simulink library "halin"  (R2021b)
settings: Solver=VariableStepAuto  StartTime=0.0  StopTime=10.0  RelTol=1e-3
undefined symbols (not defined in the file): KHAL_CAN1ABM1E2E_flg, KHAL_CAN1EPB1E2E_flg, KHAL_CAN1EPS1E2E_flg, KHAL_CAN1ESC1E2E_flg, KHAL_CAN1ESC5E2E_flg, KHAL_CAN3BMS1E2E_flg, KHAL_CAN3BMS6E2E_flg, KHAL_CAN3CCU1E2E_flg, KHAL_CAN3CCU2E2E_flg, KHAL_CAN3MCUNF1E2E_flg, KHAL_CAN3MCUNR1E2E_flg, KHAL_CAN3Shifter1E2E_flg, KHAL_CAN3Shifter2E2E_flg, KHAL_CAN6FCM2E2E_flg, KHAL_CAN6FCM4E2E_flg, TRUE
libraries: simulink x645, FVT_lib x207, hcu_lib x59
(part 17 of 23)

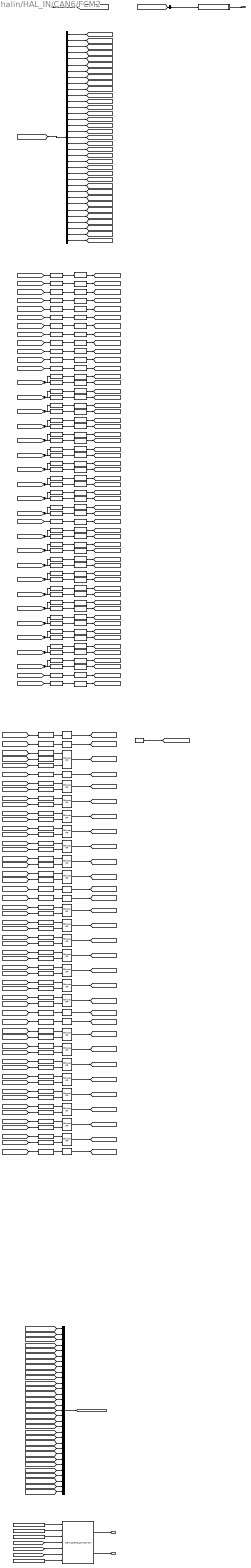
== system halin/HAL_IN/CAN6/FCM2 ==
  DT_CAN6_SG_FCM2 : Inport
  0x55 : Constant  Value=0x55
  0xEB : Constant  Value=0xEB
  ADBVehDst1Val : Subsystem
  BitwiseAND{,1..54} (55 alike) : simulink/Logic and Bit Operations/Bitwise Operator  logicop=AND  UseBitMask=on  BitMask=0xFF  BitMaskRealWorld=Stored Integer
  BitwiseOR{,1,3,11..12,20..21,30} (8 alike) : simulink/Logic and Bit Operations/Bitwise Operator  logicop=OR  UseBitMask=off  BitMask=bin2dec('11011001')  BitMaskRealWorld=Stored Integer
  BitwiseOR{4..10,13..19,22..29} (22 alike) : simulink/Logic and Bit Operations/Bitwise Operator  logicop=OR  UseBitMask=off  NumInputPorts=2  BitMask=bin2dec('11011001')  BitMaskRealWorld=Stored Integer
  BitwiseOR2 : simulink/Logic and Bit Operations/Bitwise Operator  logicop=OR  UseBitMask=off  NumInputPorts=3  BitMask=bin2dec('11011001')  BitMaskRealWorld=Stored Integer
  DDM_CS&RC_Comparison : FVT_lib/hal/DDM_CS&RC_Comparison  MsgCycleTime=50
  Data Type Conversion{,1..54} (55 alike) : DataTypeConversion  OutDataTypeStr=uint8
  KHAL_CAN6FCM2E2E_flg : Constant  Value=KHAL_CAN6FCM2E2E_flg
  LeftShift : ArithShift  BitShiftNumber=6  BitShiftDirection=Left
  LeftShift{1,3,5,7,9,11,13..14} (8 alike) : ArithShift  BitShiftDirection=Left
  LeftShift{2,4,6,8,10} (5 alike) : ArithShift  BitShiftNumber=4  BitShiftDirection=Left
  LeftShift12 : ArithShift  BitShiftNumber=2  BitShiftDirection=Left
  MessageRollingCounter : FVT_lib/hal/MessageRollingCounter  CounterMAX=14  task_time_ms=5  msg_time_ms=50
  Mux : Mux  Inputs=31
  RightShift : ArithShift  BitShiftNumber=3
  RightShift1 : ArithShift  BitShiftNumber=-5
  RightShift10 : ArithShift  BitShiftNumber=1
  RightShift11 : ArithShift  BitShiftNumber=-7
  RightShift12 : ArithShift  BitShiftNumber=3
  RightShift13 : ArithShift  BitShiftNumber=-5
  RightShift14 : ArithShift  BitShiftNumber=5
  RightShift15 : ArithShift  BitShiftNumber=-3
  RightShift16 : ArithShift  BitShiftNumber=7
  RightShift17 : ArithShift  BitShiftNumber=-1
  RightShift18 : ArithShift  BitShiftNumber=1
  RightShift19 : ArithShift  BitShiftNumber=-7
  RightShift2 : ArithShift  BitShiftNumber=1
  RightShift20 : ArithShift  BitShiftNumber=4
  RightShift21 : ArithShift  BitShiftNumber=-4
  RightShift22 : ArithShift  BitShiftNumber=2
  RightShift23 : ArithShift  BitShiftNumber=-6
  RightShift24 : ArithShift  BitShiftNumber=4
  RightShift25 : ArithShift  BitShiftNumber=-4
  RightShift26 : ArithShift  BitShiftNumber=6
  RightShift27 : ArithShift  BitShiftNumber=-2
  RightShift28 : ArithShift  BitShiftNumber=8
  RightShift29 : ArithShift
  RightShift3 : ArithShift  BitShiftNumber=-7
  RightShift30 : ArithShift  BitShiftNumber=2
  RightShift31 : ArithShift  BitShiftNumber=-6
  RightShift32 : ArithShift  BitShiftNumber=4
  RightShift33 : ArithShift  BitShiftNumber=-4
  RightShift34 : ArithShift  BitShiftNumber=6
  RightShift35 : ArithShift  BitShiftNumber=-2
  RightShift36 : ArithShift  BitShiftNumber=8
  RightShift37 : ArithShift
  RightShift38 : ArithShift  BitShiftNumber=2
  RightShift39 : ArithShift  BitShiftNumber=-6
  RightShift4 : ArithShift  BitShiftNumber=3
  RightShift5 : ArithShift  BitShiftNumber=-5
  RightShift6 : ArithShift  BitShiftNumber=5
  RightShift7 : ArithShift  BitShiftNumber=-3
  RightShift8 : ArithShift  BitShiftNumber=7
  RightShift9 : ArithShift  BitShiftNumber=-1
  bus_selector : BusSelector  OutputSignals=CAN6_ADB_FR_CMR_Sta,CAN6_ADB_ILLAmbtSta,CAN6_ADB_VehDst10Val,CAN6_ADB_VehDst1Val,CAN6_ADB_VehDst2Val,CAN6_ADB_VehDst3Val,CAN6_ADB_VehDst4Val,CAN6_ADB_VehDst5Val,CAN6_ADB_VehDst6Val,CAN6_ADB_VehDst7Val,CAN6_ADB_VehDst8Val,CAN6_ADB_VehDst9Val,CAN6_ADB_VehLtAngl10Val,CAN6_ADB_VehLtAngl1Val,CAN6_ADB_VehLtAngl2Val,CAN6_ADB_VehLtAngl3Val,CAN6_ADB_VehLtAngl4Val,CAN6_ADB_VehLtAngl5Val,CAN6_ADB_VehLtAngl6Val,CAN6_ADB_VehLtAngl7Val,CAN6_ADB_VehLtAngl8Val,CAN6_ADB_VehLtAngl9Val,CAN6_ADB_VehNumVal,CAN6_ADB_VehRtAngl10Val,CAN6_ADB_VehRtAngl1Val,CAN6_ADB_VehRtAngl2Val,CAN6_ADB_VehRtAngl3Val,CAN6_ADB_VehRtAngl4Val,CAN6_ADB_VehRtAngl5Val,CAN6_ADB_VehRtAngl6Val,CAN6_ADB_VehRtAngl7Val,CAN6_ADB_VehRtAngl8Val,CAN6_ADB_VehRtAngl9Val,CAN6_FCM2_Checksum,CAN6_FCM2_LifeCount
  bus_selector1 : BusSelector  OutputSignals=CAN6_ADB_VehDst1Val
  constant : Constant  Value=0x0  OutDataTypeStr=uint8
  VHAL_FCM2CSErr_flg : Outport
  VHAL_FCM2RCErr_flg : Outport  Port=2
  VHAL_ADBVehDst1Val_enum : Outport  Port=3
  wires:
  DT_CAN6_SG_FCM2/1 -> [DT_CAN6_SG_FCM2]
  [DT_CAN6_SG_FCM2] -> bus_selector/1
  bus_selector/1 -> [CAN6_ADB_FR_CMR_Sta]  "<CAN6_ADB_FR_CMR_Sta>"
  [CAN6_ADB_FR_CMR_Sta] -> LeftShift/1
  LeftShift/1 -> BitwiseAND/1
  BitwiseAND/1 -> [Byte_2_CAN6_ADB_FR_CMR_Sta]
  bus_selector/2 -> [CAN6_ADB_ILLAmbtSta]  "<CAN6_ADB_ILLAmbtSta>"
  [CAN6_ADB_ILLAmbtSta] -> LeftShift1/1
  LeftShift1/1 -> BitwiseAND1/1
  BitwiseAND1/1 -> [Byte_2_CAN6_ADB_ILLAmbtSta]
  bus_selector/3 -> [CAN6_ADB_VehDst10Val]  "<CAN6_ADB_VehDst10Val>"
  [CAN6_ADB_VehDst10Val] -> LeftShift2/1
  LeftShift2/1 -> BitwiseAND2/1
  BitwiseAND2/1 -> [Byte_30_CAN6_ADB_VehDst10Val]
  bus_selector/4 -> [CAN6_ADB_VehDst1Val]  "<CAN6_ADB_VehDst1Val>"
  [CAN6_ADB_VehDst1Val] -> LeftShift3/1
  LeftShift3/1 -> BitwiseAND3/1
  BitwiseAND3/1 -> [Byte_25_CAN6_ADB_VehDst1Val]
  bus_selector/5 -> [CAN6_ADB_VehDst2Val]  "<CAN6_ADB_VehDst2Val>"
  [CAN6_ADB_VehDst2Val] -> LeftShift4/1
  LeftShift4/1 -> BitwiseAND4/1
  BitwiseAND4/1 -> [Byte_26_CAN6_ADB_VehDst2Val]
  bus_selector/6 -> [CAN6_ADB_VehDst3Val]  "<CAN6_ADB_VehDst3Val>"
  [CAN6_ADB_VehDst3Val] -> LeftShift5/1
  LeftShift5/1 -> BitwiseAND5/1
  BitwiseAND5/1 -> [Byte_26_CAN6_ADB_VehDst3Val]
  bus_selector/7 -> [CAN6_ADB_VehDst4Val]  "<CAN6_ADB_VehDst4Val>"
  [CAN6_ADB_VehDst4Val] -> LeftShift6/1
  LeftShift6/1 -> BitwiseAND6/1
  BitwiseAND6/1 -> [Byte_27_CAN6_ADB_VehDst4Val]
  bus_selector/8 -> [CAN6_ADB_VehDst5Val]  "<CAN6_ADB_VehDst5Val>"
  [CAN6_ADB_VehDst5Val] -> LeftShift7/1
  LeftShift7/1 -> BitwiseAND7/1
  BitwiseAND7/1 -> [Byte_27_CAN6_ADB_VehDst5Val]
  bus_selector/9 -> [CAN6_ADB_VehDst6Val]  "<CAN6_ADB_VehDst6Val>"
  [CAN6_ADB_VehDst6Val] -> LeftShift8/1
  LeftShift8/1 -> BitwiseAND8/1
  BitwiseAND8/1 -> [Byte_28_CAN6_ADB_VehDst6Val]
  bus_selector/10 -> [CAN6_ADB_VehDst7Val]  "<CAN6_ADB_VehDst7Val>"
  [CAN6_ADB_VehDst7Val] -> LeftShift9/1
  LeftShift9/1 -> BitwiseAND9/1
  BitwiseAND9/1 -> [Byte_28_CAN6_ADB_VehDst7Val]
  bus_selector/11 -> [CAN6_ADB_VehDst8Val]  "<CAN6_ADB_VehDst8Val>"
  [CAN6_ADB_VehDst8Val] -> LeftShift10/1
  LeftShift10/1 -> BitwiseAND10/1
  BitwiseAND10/1 -> [Byte_29_CAN6_ADB_VehDst8Val]
  bus_selector/12 -> [CAN6_ADB_VehDst9Val]  "<CAN6_ADB_VehDst9Val>"
  [CAN6_ADB_VehDst9Val] -> LeftShift11/1
  LeftShift11/1 -> BitwiseAND11/1
  BitwiseAND11/1 -> [Byte_29_CAN6_ADB_VehDst9Val]
  bus_selector/13 -> [CAN6_ADB_VehLtAngl10Val]  "<CAN6_ADB_VehLtAngl10Val>"
  [CAN6_ADB_VehLtAngl10Val] -> RightShift/1, RightShift1/1
  RightShift/1 -> BitwiseAND12/1
  BitwiseAND12/1 -> [Byte_23_CAN6_ADB_VehLtAngl10Val]
  RightShift1/1 -> BitwiseAND13/1
  BitwiseAND13/1 -> [Byte_24_CAN6_ADB_VehLtAngl10Val]
  bus_selector/14 -> [CAN6_ADB_VehLtAngl1Val]  "<CAN6_ADB_VehLtAngl1Val>"
  [CAN6_ADB_VehLtAngl1Val] -> RightShift2/1, RightShift3/1
  RightShift2/1 -> BitwiseAND14/1
  BitwiseAND14/1 -> [Byte_3_CAN6_ADB_VehLtAngl1Val]
  RightShift3/1 -> BitwiseAND15/1
  BitwiseAND15/1 -> [Byte_4_CAN6_ADB_VehLtAngl1Val]
  bus_selector/15 -> [CAN6_ADB_VehLtAngl2Val]  "<CAN6_ADB_VehLtAngl2Val>"
  [CAN6_ADB_VehLtAngl2Val] -> RightShift4/1, RightShift5/1
  RightShift4/1 -> BitwiseAND16/1
  BitwiseAND16/1 -> [Byte_5_CAN6_ADB_VehLtAngl2Val]
  RightShift5/1 -> BitwiseAND17/1
  BitwiseAND17/1 -> [Byte_6_CAN6_ADB_VehLtAngl2Val]
  bus_selector/16 -> [CAN6_ADB_VehLtAngl3Val]  "<CAN6_ADB_VehLtAngl3Val>"
  [CAN6_ADB_VehLtAngl3Val] -> RightShift6/1, RightShift7/1
  RightShift6/1 -> BitwiseAND18/1
  BitwiseAND18/1 -> [Byte_7_CAN6_ADB_VehLtAngl3Val]
  RightShift7/1 -> BitwiseAND19/1
  BitwiseAND19/1 -> [Byte_8_CAN6_ADB_VehLtAngl3Val]
  bus_selector/17 -> [CAN6_ADB_VehLtAngl4Val]  "<CAN6_ADB_VehLtAngl4Val>"
  [CAN6_ADB_VehLtAngl4Val] -> RightShift8/1, RightShift9/1
  RightShift8/1 -> BitwiseAND20/1
  BitwiseAND20/1 -> [Byte_9_CAN6_ADB_VehLtAngl4Val]
  RightShift9/1 -> BitwiseAND21/1
  BitwiseAND21/1 -> [Byte_10_CAN6_ADB_VehLtAngl4Val]
  bus_selector/18 -> [CAN6_ADB_VehLtAngl5Val]  "<CAN6_ADB_VehLtAngl5Val>"
  [CAN6_ADB_VehLtAngl5Val] -> RightShift10/1, RightShift11/1
  RightShift10/1 -> BitwiseAND22/1
  BitwiseAND22/1 -> [Byte_12_CAN6_ADB_VehLtAngl5Val]
  RightShift11/1 -> BitwiseAND23/1
  BitwiseAND23/1 -> [Byte_13_CAN6_ADB_VehLtAngl5Val]
  bus_selector/19 -> [CAN6_ADB_VehLtAngl6Val]  "<CAN6_ADB_VehLtAngl6Val>"
  [CAN6_ADB_VehLtAngl6Val] -> RightShift12/1, RightShift13/1
  RightShift12/1 -> BitwiseAND24/1
  BitwiseAND24/1 -> [Byte_14_CAN6_ADB_VehLtAngl6Val]
  RightShift13/1 -> BitwiseAND25/1
  BitwiseAND25/1 -> [Byte_15_CAN6_ADB_VehLtAngl6Val]
  bus_selector/20 -> [CAN6_ADB_VehLtAngl7Val]  "<CAN6_ADB_VehLtAngl7Val>"
  [CAN6_ADB_VehLtAngl7Val] -> RightShift14/1, RightShift15/1
  RightShift14/1 -> BitwiseAND26/1
  BitwiseAND26/1 -> [Byte_16_CAN6_ADB_VehLtAngl7Val]
  RightShift15/1 -> BitwiseAND27/1
  BitwiseAND27/1 -> [Byte_17_CAN6_ADB_VehLtAngl7Val]
  bus_selector/21 -> [CAN6_ADB_VehLtAngl8Val]  "<CAN6_ADB_VehLtAngl8Val>"
  [CAN6_ADB_VehLtAngl8Val] -> RightShift16/1, RightShift17/1
  RightShift16/1 -> BitwiseAND28/1
  BitwiseAND28/1 -> [Byte_18_CAN6_ADB_VehLtAngl8Val]
  RightShift17/1 -> BitwiseAND29/1
  BitwiseAND29/1 -> [Byte_19_CAN6_ADB_VehLtAngl8Val]
  bus_selector/22 -> [CAN6_ADB_VehLtAngl9Val]  "<CAN6_ADB_VehLtAngl9Val>"
  [CAN6_ADB_VehLtAngl9Val] -> RightShift18/1, RightShift19/1
  RightShift18/1 -> BitwiseAND30/1
  BitwiseAND30/1 -> [Byte_21_CAN6_ADB_VehLtAngl9Val]
  RightShift19/1 -> BitwiseAND31/1
  BitwiseAND31/1 -> [Byte_22_CAN6_ADB_VehLtAngl9Val]
  bus_selector/23 -> [CAN6_ADB_VehNumVal]  "<CAN6_ADB_VehNumVal>"
  [CAN6_ADB_VehNumVal] -> LeftShift12/1
  LeftShift12/1 -> BitwiseAND32/1
  BitwiseAND32/1 -> [Byte_2_CAN6_ADB_VehNumVal]
  bus_selector/24 -> [CAN6_ADB_VehRtAngl10Val]  "<CAN6_ADB_VehRtAngl10Val>"
  [CAN6_ADB_VehRtAngl10Val] -> RightShift20/1, RightShift21/1
  RightShift20/1 -> BitwiseAND33/1
  BitwiseAND33/1 -> [Byte_24_CAN6_ADB_VehRtAngl10Val]
  RightShift21/1 -> BitwiseAND34/1
  BitwiseAND34/1 -> [Byte_25_CAN6_ADB_VehRtAngl10Val]
  bus_selector/25 -> [CAN6_ADB_VehRtAngl1Val]  "<CAN6_ADB_VehRtAngl1Val>"
  [CAN6_ADB_VehRtAngl1Val] -> RightShift22/1, RightShift23/1
  RightShift22/1 -> BitwiseAND35/1
  BitwiseAND35/1 -> [Byte_4_CAN6_ADB_VehRtAngl1Val]
  RightShift23/1 -> BitwiseAND36/1
  BitwiseAND36/1 -> [Byte_5_CAN6_ADB_VehRtAngl1Val]
  bus_selector/26 -> [CAN6_ADB_VehRtAngl2Val]  "<CAN6_ADB_VehRtAngl2Val>"
  [CAN6_ADB_VehRtAngl2Val] -> RightShift24/1, RightShift25/1
  RightShift24/1 -> BitwiseAND37/1
  BitwiseAND37/1 -> [Byte_6_CAN6_ADB_VehRtAngl2Val]
  RightShift25/1 -> BitwiseAND38/1
  BitwiseAND38/1 -> [Byte_7_CAN6_ADB_VehRtAngl2Val]
  bus_selector/27 -> [CAN6_ADB_VehRtAngl3Val]  "<CAN6_ADB_VehRtAngl3Val>"
  [CAN6_ADB_VehRtAngl3Val] -> RightShift26/1, RightShift27/1
  RightShift26/1 -> BitwiseAND39/1
  BitwiseAND39/1 -> [Byte_8_CAN6_ADB_VehRtAngl3Val]
  RightShift27/1 -> BitwiseAND40/1
  BitwiseAND40/1 -> [Byte_9_CAN6_ADB_VehRtAngl3Val]
  bus_selector/28 -> [CAN6_ADB_VehRtAngl4Val]  "<CAN6_ADB_VehRtAngl4Val>"
  [CAN6_ADB_VehRtAngl4Val] -> RightShift28/1, RightShift29/1
  RightShift28/1 -> BitwiseAND41/1
  BitwiseAND41/1 -> [Byte_10_CAN6_ADB_VehRtAngl4Val]
  RightShift29/1 -> BitwiseAND42/1
  BitwiseAND42/1 -> [Byte_11_CAN6_ADB_VehRtAngl4Val]
  bus_selector/29 -> [CAN6_ADB_VehRtAngl5Val]  "<CAN6_ADB_VehRtAngl5Val>"
  [CAN6_ADB_VehRtAngl5Val] -> RightShift30/1, RightShift31/1
  RightShift30/1 -> BitwiseAND43/1
  BitwiseAND43/1 -> [Byte_13_CAN6_ADB_VehRtAngl5Val]
  RightShift31/1 -> BitwiseAND44/1
  BitwiseAND44/1 -> [Byte_14_CAN6_ADB_VehRtAngl5Val]
  bus_selector/30 -> [CAN6_ADB_VehRtAngl6Val]  "<CAN6_ADB_VehRtAngl6Val>"
  [CAN6_ADB_VehRtAngl6Val] -> RightShift32/1, RightShift33/1
  RightShift32/1 -> BitwiseAND45/1
  BitwiseAND45/1 -> [Byte_15_CAN6_ADB_VehRtAngl6Val]
  RightShift33/1 -> BitwiseAND46/1
  BitwiseAND46/1 -> [Byte_16_CAN6_ADB_VehRtAngl6Val]
  bus_selector/31 -> [CAN6_ADB_VehRtAngl7Val]  "<CAN6_ADB_VehRtAngl7Val>"
  [CAN6_ADB_VehRtAngl7Val] -> RightShift34/1, RightShift35/1
  RightShift34/1 -> BitwiseAND47/1
  BitwiseAND47/1 -> [Byte_17_CAN6_ADB_VehRtAngl7Val]
  RightShift35/1 -> BitwiseAND48/1
  BitwiseAND48/1 -> [Byte_18_CAN6_ADB_VehRtAngl7Val]
  bus_selector/32 -> [CAN6_ADB_VehRtAngl8Val]  "<CAN6_ADB_VehRtAngl8Val>"
  [CAN6_ADB_VehRtAngl8Val] -> RightShift36/1, RightShift37/1
  RightShift36/1 -> BitwiseAND49/1
  BitwiseAND49/1 -> [Byte_19_CAN6_ADB_VehRtAngl8Val]
  RightShift37/1 -> BitwiseAND50/1
  BitwiseAND50/1 -> [Byte_20_CAN6_ADB_VehRtAngl8Val]
  bus_selector/33 -> [CAN6_ADB_VehRtAngl9Val]  "<CAN6_ADB_VehRtAngl9Val>"
  [CAN6_ADB_VehRtAngl9Val] -> RightShift38/1, RightShift39/1
  RightShift38/1 -> BitwiseAND51/1
  BitwiseAND51/1 -> [Byte_22_CAN6_ADB_VehRtAngl9Val]
  RightShift39/1 -> BitwiseAND52/1
  BitwiseAND52/1 -> [Byte_23_CAN6_ADB_VehRtAngl9Val]
  bus_selector/34 -> [CAN6_FCM2_Checksum]  "<CAN6_FCM2_Checksum>"
  [CAN6_FCM2_Checksum] -> LeftShift13/1
  LeftShift13/1 -> BitwiseAND53/1
  BitwiseAND53/1 -> [Byte_0_CAN6_FCM2_Checksum]
  bus_selector/35 -> [CAN6_FCM2_LifeCount]  "<CAN6_FCM2_LifeCount>"
  [CAN6_FCM2_LifeCount] -> LeftShift14/1
  LeftShift14/1 -> BitwiseAND54/1
  BitwiseAND54/1 -> [Byte_1_CAN6_FCM2_LifeCount]
  Data Type Conversion/1 -> BitwiseOR/1
  [Byte_0_CAN6_FCM2_Checksum] -> Data Type Conversion/1
  BitwiseOR/1 -> [Byte_0]
  Data Type Conversion1/1 -> BitwiseOR1/1
  [Byte_1_CAN6_FCM2_LifeCount] -> Data Type Conversion1/1
  BitwiseOR1/1 -> [Byte_1]
  Data Type Conversion2/1 -> BitwiseOR2/1
  [Byte_2_CAN6_ADB_FR_CMR_Sta] -> Data Type Conversion2/1
  Data Type Conversion3/1 -> BitwiseOR2/2
  [Byte_2_CAN6_ADB_ILLAmbtSta] -> Data Type Conversion3/1
  Data Type Conversion4/1 -> BitwiseOR2/3
  [Byte_2_CAN6_ADB_VehNumVal] -> Data Type Conversion4/1
  BitwiseOR2/1 -> [Byte_2]
  Data Type Conversion5/1 -> BitwiseOR3/1
  [Byte_3_CAN6_ADB_VehLtAngl1Val] -> Data Type Conversion5/1
  BitwiseOR3/1 -> [Byte_3]
  Data Type Conversion6/1 -> BitwiseOR4/1
  [Byte_4_CAN6_ADB_VehLtAngl1Val] -> Data Type Conversion6/1
  Data Type Conversion7/1 -> BitwiseOR4/2
  [Byte_4_CAN6_ADB_VehRtAngl1Val] -> Data Type Conversion7/1
  BitwiseOR4/1 -> [Byte_4]
  Data Type Conversion8/1 -> BitwiseOR5/1
  [Byte_5_CAN6_ADB_VehLtAngl2Val] -> Data Type Conversion8/1
  Data Type Conversion9/1 -> BitwiseOR5/2
  [Byte_5_CAN6_ADB_VehRtAngl1Val] -> Data Type Conversion9/1
  BitwiseOR5/1 -> [Byte_5]
  Data Type Conversion10/1 -> BitwiseOR6/1
  [Byte_6_CAN6_ADB_VehLtAngl2Val] -> Data Type Conversion10/1
  Data Type Conversion11/1 -> BitwiseOR6/2
  [Byte_6_CAN6_ADB_VehRtAngl2Val] -> Data Type Conversion11/1
  BitwiseOR6/1 -> [Byte_6]
  Data Type Conversion12/1 -> BitwiseOR7/1
  [Byte_7_CAN6_ADB_VehLtAngl3Val] -> Data Type Conversion12/1
  Data Type Conversion13/1 -> BitwiseOR7/2
  [Byte_7_CAN6_ADB_VehRtAngl2Val] -> Data Type Conversion13/1
  BitwiseOR7/1 -> [Byte_7]
  Data Type Conversion14/1 -> BitwiseOR8/1
  [Byte_8_CAN6_ADB_VehLtAngl3Val] -> Data Type Conversion14/1
  Data Type Conversion15/1 -> BitwiseOR8/2
  [Byte_8_CAN6_ADB_VehRtAngl3Val] -> Data Type Conversion15/1
  BitwiseOR8/1 -> [Byte_8]
  Data Type Conversion16/1 -> BitwiseOR9/1
  [Byte_9_CAN6_ADB_VehLtAngl4Val] -> Data Type Conversion16/1
  Data Type Conversion17/1 -> BitwiseOR9/2
  [Byte_9_CAN6_ADB_VehRtAngl3Val] -> Data Type Conversion17/1
  BitwiseOR9/1 -> [Byte_9]
  Data Type Conversion18/1 -> BitwiseOR10/1
  [Byte_10_CAN6_ADB_VehLtAngl4Val] -> Data Type Conversion18/1
  Data Type Conversion19/1 -> BitwiseOR10/2
  [Byte_10_CAN6_ADB_VehRtAngl4Val] -> Data Type Conversion19/1
  BitwiseOR10/1 -> [Byte_10]
  Data Type Conversion20/1 -> BitwiseOR11/1
  [Byte_11_CAN6_ADB_VehRtAngl4Val] -> Data Type Conversion20/1
  BitwiseOR11/1 -> [Byte_11]
  Data Type Conversion21/1 -> BitwiseOR12/1
  [Byte_12_CAN6_ADB_VehLtAngl5Val] -> Data Type Conversion21/1
  BitwiseOR12/1 -> [Byte_12]
  Data Type Conversion22/1 -> BitwiseOR13/1
  [Byte_13_CAN6_ADB_VehLtAngl5Val] -> Data Type Conversion22/1
  Data Type Conversion23/1 -> BitwiseOR13/2
  [Byte_13_CAN6_ADB_VehRtAngl5Val] -> Data Type Conversion23/1
  BitwiseOR13/1 -> [Byte_13]
  Data Type Conversion24/1 -> BitwiseOR14/1
  [Byte_14_CAN6_ADB_VehLtAngl6Val] -> Data Type Conversion24/1
  Data Type Conversion25/1 -> BitwiseOR14/2
  [Byte_14_CAN6_ADB_VehRtAngl5Val] -> Data Type Conversion25/1
  BitwiseOR14/1 -> [Byte_14]
  Data Type Conversion26/1 -> BitwiseOR15/1
  [Byte_15_CAN6_ADB_VehLtAngl6Val] -> Data Type Conversion26/1
  Data Type Conversion27/1 -> BitwiseOR15/2
  [Byte_15_CAN6_ADB_VehRtAngl6Val] -> Data Type Conversion27/1
  BitwiseOR15/1 -> [Byte_15]
  Data Type Conversion28/1 -> BitwiseOR16/1
  [Byte_16_CAN6_ADB_VehLtAngl7Val] -> Data Type Conversion28/1
  Data Type Conversion29/1 -> BitwiseOR16/2
  [Byte_16_CAN6_ADB_VehRtAngl6Val] -> Data Type Conversion29/1
  BitwiseOR16/1 -> [Byte_16]
  Data Type Conversion30/1 -> BitwiseOR17/1
  [Byte_17_CAN6_ADB_VehLtAngl7Val] -> Data Type Conversion30/1
  Data Type Conversion31/1 -> BitwiseOR17/2
  [Byte_17_CAN6_ADB_VehRtAngl7Val] -> Data Type Conversion31/1
  BitwiseOR17/1 -> [Byte_17]
  Data Type Conversion32/1 -> BitwiseOR18/1
  [Byte_18_CAN6_ADB_VehLtAngl8Val] -> Data Type Conversion32/1
  Data Type Conversion33/1 -> BitwiseOR18/2
  [Byte_18_CAN6_ADB_VehRtAngl7Val] -> Data Type Conversion33/1
  BitwiseOR18/1 -> [Byte_18]
  Data Type Conversion34/1 -> BitwiseOR19/1
  [Byte_19_CAN6_ADB_VehLtAngl8Val] -> Data Type Conversion34/1
  Data Type Conversion35/1 -> BitwiseOR19/2
  [Byte_19_CAN6_ADB_VehRtAngl8Val] -> Data Type Conversion35/1
  BitwiseOR19/1 -> [Byte_19]
  Data Type Conversion36/1 -> BitwiseOR20/1
  [Byte_20_CAN6_ADB_VehRtAngl8Val] -> Data Type Conversion36/1
  BitwiseOR20/1 -> [Byte_20]
  Data Type Conversion37/1 -> BitwiseOR21/1
  [Byte_21_CAN6_ADB_VehLtAngl9Val] -> Data Type Conversion37/1
  BitwiseOR21/1 -> [Byte_21]
  Data Type Conversion38/1 -> BitwiseOR22/1
  [Byte_22_CAN6_ADB_VehLtAngl9Val] -> Data Type Conversion38/1
  Data Type Conversion39/1 -> BitwiseOR22/2
  [Byte_22_CAN6_ADB_VehRtAngl9Val] -> Data Type Conversion39/1
  BitwiseOR22/1 -> [Byte_22]
  Data Type Conversion40/1 -> BitwiseOR23/1
  [Byte_23_CAN6_ADB_VehLtAngl10Val] -> Data Type Conversion40/1
  Data Type Conversion41/1 -> BitwiseOR23/2
  [Byte_23_CAN6_ADB_VehRtAngl9Val] -> Data Type Conversion41/1
  BitwiseOR23/1 -> [Byte_23]
  Data Type Conversion42/1 -> BitwiseOR24/1
  [Byte_24_CAN6_ADB_VehLtAngl10Val] -> Data Type Conversion42/1
  Data Type Conversion43/1 -> BitwiseOR24/2
  [Byte_24_CAN6_ADB_VehRtAngl10Val] -> Data Type Conversion43/1
  BitwiseOR24/1 -> [Byte_24]
  Data Type Conversion44/1 -> BitwiseOR25/1
  [Byte_25_CAN6_ADB_VehDst1Val] -> Data Type Conversion44/1
  Data Type Conversion45/1 -> BitwiseOR25/2
  [Byte_25_CAN6_ADB_VehRtAngl10Val] -> Data Type Conversion45/1
  BitwiseOR25/1 -> [Byte_25]
  Data Type Conversion46/1 -> BitwiseOR26/1
  [Byte_26_CAN6_ADB_VehDst2Val] -> Data Type Conversion46/1
  Data Type Conversion47/1 -> BitwiseOR26/2
  [Byte_26_CAN6_ADB_VehDst3Val] -> Data Type Conversion47/1
  BitwiseOR26/1 -> [Byte_26]
  Data Type Conversion48/1 -> BitwiseOR27/1
  [Byte_27_CAN6_ADB_VehDst4Val] -> Data Type Conversion48/1
  Data Type Conversion49/1 -> BitwiseOR27/2
  [Byte_27_CAN6_ADB_VehDst5Val] -> Data Type Conversion49/1
  BitwiseOR27/1 -> [Byte_27]
  Data Type Conversion50/1 -> BitwiseOR28/1
  [Byte_28_CAN6_ADB_VehDst6Val] -> Data Type Conversion50/1
  Data Type Conversion51/1 -> BitwiseOR28/2
  [Byte_28_CAN6_ADB_VehDst7Val] -> Data Type Conversion51/1
  BitwiseOR28/1 -> [Byte_28]
  Data Type Conversion52/1 -> BitwiseOR29/1
  [Byte_29_CAN6_ADB_VehDst8Val] -> Data Type Conversion52/1
  Data Type Conversion53/1 -> BitwiseOR29/2
  [Byte_29_CAN6_ADB_VehDst9Val] -> Data Type Conversion53/1
  BitwiseOR29/1 -> [Byte_29]
  Data Type Conversion54/1 -> BitwiseOR30/1
  [Byte_30_CAN6_ADB_VehDst10Val] -> Data Type Conversion54/1
  BitwiseOR30/1 -> [Byte_30]
  constant/1 -> [Byte_31]
  [Byte_1] -> Mux/1
  [Byte_2] -> Mux/2
  [Byte_3] -> Mux/3
  [Byte_4] -> Mux/4
  [Byte_5] -> Mux/5
  [Byte_6] -> Mux/6
  [Byte_7] -> Mux/7
  [Byte_8] -> Mux/8
  [Byte_9] -> Mux/9
  [Byte_10] -> Mux/10
  [Byte_11] -> Mux/11
  [Byte_12] -> Mux/12
  [Byte_13] -> Mux/13
  [Byte_14] -> Mux/14
  [Byte_15] -> Mux/15
  [Byte_16] -> Mux/16
  [Byte_17] -> Mux/17
  [Byte_18] -> Mux/18
  [Byte_19] -> Mux/19
  [Byte_20] -> Mux/20
  [Byte_21] -> Mux/21
  [Byte_22] -> Mux/22
  [Byte_23] -> Mux/23
  [Byte_24] -> Mux/24
  [Byte_25] -> Mux/25
  [Byte_26] -> Mux/26
  [Byte_27] -> Mux/27
  [Byte_28] -> Mux/28
  [Byte_29] -> Mux/29
  [Byte_30] -> Mux/30
  [Byte_31] -> Mux/31
  Mux/1 -> [VHAL_CAN6FCM2noCS_raw]
  KHAL_CAN6FCM2E2E_flg/1 -> DDM_CS&RC_Comparison/1
  0x55/1 -> DDM_CS&RC_Comparison/2
  0xEB/1 -> DDM_CS&RC_Comparison/3
  [VHAL_CAN6FCM2noCS_raw] -> DDM_CS&RC_Comparison/4
  [Byte_0] -> DDM_CS&RC_Comparison/5
  [RC_ECU] -> DDM_CS&RC_Comparison/6
  MessageRollingCounter/1 -> DDM_CS&RC_Comparison/7
  DDM_CS&RC_Comparison/1 -> VHAL_FCM2CSErr_flg/1
  DDM_CS&RC_Comparison/2 -> VHAL_FCM2RCErr_flg/1
  [DT_CAN6_SG_FCM2] -> bus_selector1/1
  bus_selector1/1 -> ADBVehDst1Val/1(ADB_VehDst1Val)  "<CAN6_ADB_VehDst1Val>"
  ADBVehDst1Val/1(VHAL_ADBVehDst1Val_enum) -> VHAL_ADBVehDst1Val_enum/1

== system halin/HAL_IN/CAN6/FCM3 ==
  DT_CAN6_SG_FCM3 : Inport
  MELaneCurvDervLt : Subsystem
  MELaneCurvDervLt2 : Subsystem
  MELaneCurvDervRt : Subsystem
  MELaneCurvDervRt2 : Subsystem
  MELaneCurvLt : Subsystem
  MELaneCurvLt2 : Subsystem
  MELaneCurvRt : Subsystem
  MELaneCurvRt2 : Subsystem
  MELaneHeadAngLt : Subsystem
  MELaneHeadAngLt2 : Subsystem
  MELaneHeadAngRt : Subsystem
  MELaneHeadAngRt2 : Subsystem
  MELanePosLt : Subsystem
  MELanePosLt2 : Subsystem
  MELanePosRt : Subsystem
  MELanePosRt2 : Subsystem
  bus_selector : BusSelector  OutputSignals=CAN6_ME_Lane_CurvDervLt
  bus_selector1 : BusSelector  OutputSignals=CAN6_ME_Lane_CurvDervLt2
  bus_selector10 : BusSelector  OutputSignals=CAN6_ME_Lane_HeadAngRt
  bus_selector11 : BusSelector  OutputSignals=CAN6_ME_Lane_HeadAngRt2
  bus_selector12 : BusSelector  OutputSignals=CAN6_ME_Lane_PosLt
  bus_selector13 : BusSelector  OutputSignals=CAN6_ME_Lane_PosLt2
  bus_selector14 : BusSelector  OutputSignals=CAN6_ME_Lane_PosRt
  bus_selector15 : BusSelector  OutputSignals=CAN6_ME_Lane_PosRt2
  bus_selector2 : BusSelector  OutputSignals=CAN6_ME_Lane_CurvDervRt
  bus_selector3 : BusSelector  OutputSignals=CAN6_ME_Lane_CurvDervRt2
  bus_selector4 : BusSelector  OutputSignals=CAN6_ME_Lane_CurvLt
  bus_selector5 : BusSelector  OutputSignals=CAN6_ME_Lane_CurvLt2
  bus_selector6 : BusSelector  OutputSignals=CAN6_ME_Lane_CurvRt
  bus_selector7 : BusSelector  OutputSignals=CAN6_ME_Lane_CurvRt2
  bus_selector8 : BusSelector  OutputSignals=CAN6_ME_Lane_HeadAngLt
  bus_selector9 : BusSelector  OutputSignals=CAN6_ME_Lane_HeadAngLt2
  VHAL_MELaneCurvDervLt_raw32 : Outport
  VHAL_MELaneCurvDervLt2_raw32 : Outport  Port=2
  VHAL_MELaneCurvDervRt_raw32 : Outport  Port=3
  VHAL_MELaneCurvDervRt2_raw32 : Outport  Port=4
  VHAL_MELaneCurvLt_raw32 : Outport  Port=5
  VHAL_MELaneCurvLt2_raw32 : Outport  Port=6
  VHAL_MELaneCurvRt_raw32 : Outport  Port=7
  VHAL_MELaneCurvRt2_raw32 : Outport  Port=8
  VHAL_MELaneHeadAngLt_radians : Outport  Port=9
  VHAL_MELaneHeadAngLt2_radians : Outport  Port=10
  VHAL_MELaneHeadAngRt_radians : Outport  Port=11
  VHAL_MELaneHeadAngRt2_radians : Outport  Port=12
  VHAL_MELanePosLt_m : Outport  Port=13
  VHAL_MELanePosLt2_m : Outport  Port=14
  VHAL_MELanePosRt_m : Outport  Port=15
  VHAL_MELanePosRt2_m : Outport  Port=16
  wires:
  DT_CAN6_SG_FCM3/1 -> [DT_CAN6_SG_FCM3]
  [DT_CAN6_SG_FCM3] -> bus_selector/1
  bus_selector/1 -> MELaneCurvDervLt/1(ME_Lane_CurvDervLt)  "<CAN6_ME_Lane_CurvDervLt>"
  MELaneCurvDervLt/1(VHAL_MELaneCurvDervLt_raw32) -> VHAL_MELaneCurvDervLt_raw32/1
  [DT_CAN6_SG_FCM3] -> bus_selector1/1
  bus_selector1/1 -> MELaneCurvDervLt2/1(ME_Lane_CurvDervLt2)  "<CAN6_ME_Lane_CurvDervLt2>"
  MELaneCurvDervLt2/1(VHAL_MELaneCurvDervLt2_raw32) -> VHAL_MELaneCurvDervLt2_raw32/1
  [DT_CAN6_SG_FCM3] -> bus_selector2/1
  bus_selector2/1 -> MELaneCurvDervRt/1(ME_Lane_CurvDervRt)  "<CAN6_ME_Lane_CurvDervRt>"
  MELaneCurvDervRt/1(VHAL_MELaneCurvDervRt_raw32) -> VHAL_MELaneCurvDervRt_raw32/1
  [DT_CAN6_SG_FCM3] -> bus_selector3/1
  bus_selector3/1 -> MELaneCurvDervRt2/1(ME_Lane_CurvDervRt2)  "<CAN6_ME_Lane_CurvDervRt2>"
  MELaneCurvDervRt2/1(VHAL_MELaneCurvDervRt2_raw32) -> VHAL_MELaneCurvDervRt2_raw32/1
  [DT_CAN6_SG_FCM3] -> bus_selector4/1
  bus_selector4/1 -> MELaneCurvLt/1(ME_Lane_CurvLt)  "<CAN6_ME_Lane_CurvLt>"
  MELaneCurvLt/1(VHAL_MELaneCurvLt_raw32) -> VHAL_MELaneCurvLt_raw32/1
  [DT_CAN6_SG_FCM3] -> bus_selector5/1
  bus_selector5/1 -> MELaneCurvLt2/1(ME_Lane_CurvLt2)  "<CAN6_ME_Lane_CurvLt2>"
  MELaneCurvLt2/1(VHAL_MELaneCurvLt2_raw32) -> VHAL_MELaneCurvLt2_raw32/1
  [DT_CAN6_SG_FCM3] -> bus_selector6/1
  bus_selector6/1 -> MELaneCurvRt/1(ME_Lane_CurvRt)  "<CAN6_ME_Lane_CurvRt>"
  MELaneCurvRt/1(VHAL_MELaneCurvRt_raw32) -> VHAL_MELaneCurvRt_raw32/1
  [DT_CAN6_SG_FCM3] -> bus_selector7/1
  bus_selector7/1 -> MELaneCurvRt2/1(ME_Lane_CurvRt2)  "<CAN6_ME_Lane_CurvRt2>"
  MELaneCurvRt2/1(VHAL_MELaneCurvRt2_raw32) -> VHAL_MELaneCurvRt2_raw32/1
  [DT_CAN6_SG_FCM3] -> bus_selector8/1
  bus_selector8/1 -> MELaneHeadAngLt/1(ME_Lane_HeadAngLt)  "<CAN6_ME_Lane_HeadAngLt>"
  MELaneHeadAngLt/1(VHAL_MELaneHeadAngLt_radians) -> VHAL_MELaneHeadAngLt_radians/1
  [DT_CAN6_SG_FCM3] -> bus_selector9/1
  bus_selector9/1 -> MELaneHeadAngLt2/1(ME_Lane_HeadAngLt2)  "<CAN6_ME_Lane_HeadAngLt2>"
  MELaneHeadAngLt2/1(VHAL_MELaneHeadAngLt2_radians) -> VHAL_MELaneHeadAngLt2_radians/1
  [DT_CAN6_SG_FCM3] -> bus_selector10/1
  bus_selector10/1 -> MELaneHeadAngRt/1(ME_Lane_HeadAngRt)  "<CAN6_ME_Lane_HeadAngRt>"
  MELaneHeadAngRt/1(VHAL_MELaneHeadAngRt_radians) -> VHAL_MELaneHeadAngRt_radians/1
  [DT_CAN6_SG_FCM3] -> bus_selector11/1
  bus_selector11/1 -> MELaneHeadAngRt2/1(ME_Lane_HeadAngRt2)  "<CAN6_ME_Lane_HeadAngRt2>"
  MELaneHeadAngRt2/1(VHAL_MELaneHeadAngRt2_radians) -> VHAL_MELaneHeadAngRt2_radians/1
  [DT_CAN6_SG_FCM3] -> bus_selector12/1
  bus_selector12/1 -> MELanePosLt/1(ME_Lane_PosLt)  "<CAN6_ME_Lane_PosLt>"
  MELanePosLt/1(VHAL_MELanePosLt_m) -> VHAL_MELanePosLt_m/1
  [DT_CAN6_SG_FCM3] -> bus_selector13/1
  bus_selector13/1 -> MELanePosLt2/1(ME_Lane_PosLt2)  "<CAN6_ME_Lane_PosLt2>"
  MELanePosLt2/1(VHAL_MELanePosLt2_m) -> VHAL_MELanePosLt2_m/1
  [DT_CAN6_SG_FCM3] -> bus_selector14/1
  bus_selector14/1 -> MELanePosRt/1(ME_Lane_PosRt)  "<CAN6_ME_Lane_PosRt>"
  MELanePosRt/1(VHAL_MELanePosRt_m) -> VHAL_MELanePosRt_m/1
  [DT_CAN6_SG_FCM3] -> bus_selector15/1
  bus_selector15/1 -> MELanePosRt2/1(ME_Lane_PosRt2)  "<CAN6_ME_Lane_PosRt2>"
  MELanePosRt2/1(VHAL_MELanePosRt2_m) -> VHAL_MELanePosRt2_m/1

== system halin/HAL_IN/CAN6/FCM4 ==
  DT_CAN6_SG_FCM4 : Inport
  0xB1 : Constant  Value=0xB5
  0xB5 : Constant  Value=0xB5
  ADASAngCtrlTqWeightGain : Subsystem
  ADASDesStrWhlAngCtrlCmd : Subsystem
  ADASDrvInputTqBoostAct : Subsystem
  ADASDrvInputTqBoostGain : Subsystem
  ADASMaxAngCtrlOutTqLimit : Subsystem
  ADASStrWhlAngCtrlStatus : Subsystem
  BitwiseAND{,1..9} (10 alike) : simulink/Logic and Bit Operations/Bitwise Operator  logicop=AND  UseBitMask=on  BitMask=0xFF  BitMaskRealWorld=Stored Integer
  BitwiseOR{,1..2,4..7} (7 alike) : simulink/Logic and Bit Operations/Bitwise Operator  logicop=OR  UseBitMask=off  BitMask=bin2dec('11011001')  BitMaskRealWorld=Stored Integer
  BitwiseOR3 : simulink/Logic and Bit Operations/Bitwise Operator  logicop=OR  UseBitMask=off  NumInputPorts=3  BitMask=bin2dec('11011001')  BitMaskRealWorld=Stored Integer
  DDM_CS&RC_Comparison : FVT_lib/hal/DDM_CS&RC_Comparison  MsgCycleTime=10
  Data Type Conversion{,1..9} (10 alike) : DataTypeConversion  OutDataTypeStr=uint8
  KHAL_CAN6FCM4E2E_flg : Constant  Value=KHAL_CAN6FCM4E2E_flg
  LeftShift{,2,4..5} (4 alike) : ArithShift  BitShiftDirection=Left
  LeftShift1 : ArithShift  BitShiftNumber=5  BitShiftDirection=Left
  LeftShift3 : ArithShift  BitShiftNumber=6  BitShiftDirection=Left
  MessageRollingCounter : FVT_lib/hal/MessageRollingCounter  CounterMAX=14  task_time_ms=5  msg_time_ms=10
  Mux : Mux  Inputs=31
  RightShift : ArithShift  BitShiftNumber=8
  RightShift1 : ArithShift
  RightShift2 : ArithShift  BitShiftNumber=1
  RightShift3 : ArithShift  BitShiftNumber=-7
  bus_selector : BusSelector  OutputSignals=CAN6_ADAS_AngCtrlTqWeightGain,CAN6_ADAS_DesStrWhlAngCtrlCmd,CAN6_ADAS_DrvInputTqBoostAct,CAN6_ADAS_DrvInputTqBoostGain,CAN6_ADAS_MaxAngCtrlOutTqLimit,CAN6_ADAS_StrWhlAngCtrlStatus,CAN6_FCM4_Checksum,CAN6_FCM4_LifeCount
  bus_selector1 : BusSelector  OutputSignals=CAN6_ADAS_AngCtrlTqWeightGain
  bus_selector2 : BusSelector  OutputSignals=CAN6_ADAS_DesStrWhlAngCtrlCmd
  bus_selector3 : BusSelector  OutputSignals=CAN6_ADAS_DrvInputTqBoostAct
  bus_selector4 : BusSelector  OutputSignals=CAN6_ADAS_DrvInputTqBoostGain
  bus_selector5 : BusSelector  OutputSignals=CAN6_ADAS_MaxAngCtrlOutTqLimit
  bus_selector6 : BusSelector  OutputSignals=CAN6_ADAS_StrWhlAngCtrlStatus
  constant{,1..23} (24 alike) : Constant  Value=0x0  OutDataTypeStr=uint8
  VHAL_FCM4CSErr_flg : Outport
  VHAL_FCM4RCErr_flg : Outport  Port=2
  VHAL_ADASAngCtrlTqWeightGain_pct : Outport  Port=3
  VHAL_ADASDesStrWhlAngCtrlCmd_Deg : Outport  Port=4
  VHAL_ADASDrvInputTqBoostAct_flg : Outport  Port=5
  VHAL_ADASDrvInputTqBoostGain_pct : Outport  Port=6
  VHAL_ADASMaxAngCtrlOutTqLimit_Nm : Outport  Port=7
  VHAL_ADASStrWhlAngCtrlStatus_flg : Outport  Port=8
  wires:
  DT_CAN6_SG_FCM4/1 -> [DT_CAN6_SG_FCM4]
  [DT_CAN6_SG_FCM4] -> bus_selector/1
  bus_selector/1 -> [CAN6_ADAS_AngCtrlTqWeightGain]  "<CAN6_ADAS_AngCtrlTqWeightGain>"
  [CAN6_ADAS_AngCtrlTqWeightGain] -> LeftShift/1
  LeftShift/1 -> BitwiseAND/1
  BitwiseAND/1 -> [Byte_5_CAN6_ADAS_AngCtrlTqWeightGain]
  bus_selector/2 -> [CAN6_ADAS_DesStrWhlAngCtrlCmd]  "<CAN6_ADAS_DesStrWhlAngCtrlCmd>"
  [CAN6_ADAS_DesStrWhlAngCtrlCmd] -> RightShift/1, RightShift1/1
  RightShift/1 -> BitwiseAND1/1
  BitwiseAND1/1 -> [Byte_6_CAN6_ADAS_DesStrWhlAngCtrlCmd]
  RightShift1/1 -> BitwiseAND2/1
  BitwiseAND2/1 -> [Byte_7_CAN6_ADAS_DesStrWhlAngCtrlCmd]
  bus_selector/3 -> [CAN6_ADAS_DrvInputTqBoostAct]  "<CAN6_ADAS_DrvInputTqBoostAct>"
  [CAN6_ADAS_DrvInputTqBoostAct] -> LeftShift1/1
  LeftShift1/1 -> BitwiseAND3/1
  BitwiseAND3/1 -> [Byte_3_CAN6_ADAS_DrvInputTqBoostAct]
  bus_selector/4 -> [CAN6_ADAS_DrvInputTqBoostGain]  "<CAN6_ADAS_DrvInputTqBoostGain>"
  [CAN6_ADAS_DrvInputTqBoostGain] -> LeftShift2/1
  LeftShift2/1 -> BitwiseAND4/1
  BitwiseAND4/1 -> [Byte_4_CAN6_ADAS_DrvInputTqBoostGain]
  bus_selector/5 -> [CAN6_ADAS_MaxAngCtrlOutTqLimit]  "<CAN6_ADAS_MaxAngCtrlOutTqLimit>"
  [CAN6_ADAS_MaxAngCtrlOutTqLimit] -> RightShift2/1, RightShift3/1
  RightShift2/1 -> BitwiseAND5/1
  BitwiseAND5/1 -> [Byte_2_CAN6_ADAS_MaxAngCtrlOutTqLimit]
  RightShift3/1 -> BitwiseAND6/1
  BitwiseAND6/1 -> [Byte_3_CAN6_ADAS_MaxAngCtrlOutTqLimit]
  bus_selector/6 -> [CAN6_ADAS_StrWhlAngCtrlStatus]  "<CAN6_ADAS_StrWhlAngCtrlStatus>"
  [CAN6_ADAS_StrWhlAngCtrlStatus] -> LeftShift3/1
  LeftShift3/1 -> BitwiseAND7/1
  BitwiseAND7/1 -> [Byte_3_CAN6_ADAS_StrWhlAngCtrlStatus]
  bus_selector/7 -> [CAN6_FCM4_Checksum]  "<CAN6_FCM4_Checksum>"
  [CAN6_FCM4_Checksum] -> LeftShift4/1
  LeftShift4/1 -> BitwiseAND8/1
  BitwiseAND8/1 -> [Byte_0_CAN6_FCM4_Checksum]
  bus_selector/8 -> [CAN6_FCM4_LifeCount]  "<CAN6_FCM4_LifeCount>"
  [CAN6_FCM4_LifeCount] -> LeftShift5/1
  LeftShift5/1 -> BitwiseAND9/1
  BitwiseAND9/1 -> [Byte_1_CAN6_FCM4_LifeCount]
  Data Type Conversion/1 -> BitwiseOR/1
  [Byte_0_CAN6_FCM4_Checksum] -> Data Type Conversion/1
  BitwiseOR/1 -> [Byte_0]
  Data Type Conversion1/1 -> BitwiseOR1/1
  [Byte_1_CAN6_FCM4_LifeCount] -> Data Type Conversion1/1
  BitwiseOR1/1 -> [Byte_1]
  Data Type Conversion2/1 -> BitwiseOR2/1
  [Byte_2_CAN6_ADAS_MaxAngCtrlOutTqLimit] -> Data Type Conversion2/1
  BitwiseOR2/1 -> [Byte_2]
  Data Type Conversion3/1 -> BitwiseOR3/1
  [Byte_3_CAN6_ADAS_DrvInputTqBoostAct] -> Data Type Conversion3/1
  Data Type Conversion4/1 -> BitwiseOR3/2
  [Byte_3_CAN6_ADAS_MaxAngCtrlOutTqLimit] -> Data Type Conversion4/1
  Data Type Conversion5/1 -> BitwiseOR3/3
  [Byte_3_CAN6_ADAS_StrWhlAngCtrlStatus] -> Data Type Conversion5/1
  BitwiseOR3/1 -> [Byte_3]
  Data Type Conversion6/1 -> BitwiseOR4/1
  [Byte_4_CAN6_ADAS_DrvInputTqBoostGain] -> Data Type Conversion6/1
  BitwiseOR4/1 -> [Byte_4]
  Data Type Conversion7/1 -> BitwiseOR5/1
  [Byte_5_CAN6_ADAS_AngCtrlTqWeightGain] -> Data Type Conversion7/1
  BitwiseOR5/1 -> [Byte_5]
  Data Type Conversion8/1 -> BitwiseOR6/1
  [Byte_6_CAN6_ADAS_DesStrWhlAngCtrlCmd] -> Data Type Conversion8/1
  BitwiseOR6/1 -> [Byte_6]
  Data Type Conversion9/1 -> BitwiseOR7/1
  [Byte_7_CAN6_ADAS_DesStrWhlAngCtrlCmd] -> Data Type Conversion9/1
  BitwiseOR7/1 -> [Byte_7]
  constant/1 -> [Byte_8]
  constant1/1 -> [Byte_9]
  constant2/1 -> [Byte_10]
  constant3/1 -> [Byte_11]
  constant4/1 -> [Byte_12]
  constant5/1 -> [Byte_13]
  constant6/1 -> [Byte_14]
  constant7/1 -> [Byte_15]
  constant8/1 -> [Byte_16]
  constant9/1 -> [Byte_17]
  constant10/1 -> [Byte_18]
  constant11/1 -> [Byte_19]
  constant12/1 -> [Byte_20]
  constant13/1 -> [Byte_21]
  constant14/1 -> [Byte_22]
  constant15/1 -> [Byte_23]
  constant16/1 -> [Byte_24]
  constant17/1 -> [Byte_25]
  constant18/1 -> [Byte_26]
  constant19/1 -> [Byte_27]
  constant20/1 -> [Byte_28]
  constant21/1 -> [Byte_29]
  constant22/1 -> [Byte_30]
  constant23/1 -> [Byte_31]
  [Byte_1] -> Mux/1
  [Byte_2] -> Mux/2
  [Byte_3] -> Mux/3
  [Byte_4] -> Mux/4
  [Byte_5] -> Mux/5
  [Byte_6] -> Mux/6
  [Byte_7] -> Mux/7
  [Byte_8] -> Mux/8
  [Byte_9] -> Mux/9
  [Byte_10] -> Mux/10
  [Byte_11] -> Mux/11
  [Byte_12] -> Mux/12
  [Byte_13] -> Mux/13
  [Byte_14] -> Mux/14
  [Byte_15] -> Mux/15
  [Byte_16] -> Mux/16
  [Byte_17] -> Mux/17
  [Byte_18] -> Mux/18
  [Byte_19] -> Mux/19
  [Byte_20] -> Mux/20
  [Byte_21] -> Mux/21
  [Byte_22] -> Mux/22
  [Byte_23] -> Mux/23
  [Byte_24] -> Mux/24
  [Byte_25] -> Mux/25
  [Byte_26] -> Mux/26
  [Byte_27] -> Mux/27
  [Byte_28] -> Mux/28
  [Byte_29] -> Mux/29
  [Byte_30] -> Mux/30
  [Byte_31] -> Mux/31
  Mux/1 -> [VHAL_CAN6FCM4noCS_raw]
  KHAL_CAN6FCM4E2E_flg/1 -> DDM_CS&RC_Comparison/1
  0xB5/1 -> DDM_CS&RC_Comparison/2
  0xB1/1 -> DDM_CS&RC_Comparison/3
  [VHAL_CAN6FCM4noCS_raw] -> DDM_CS&RC_Comparison/4
  [Byte_0] -> DDM_CS&RC_Comparison/5
  [RC_ECU] -> DDM_CS&RC_Comparison/6
  MessageRollingCounter/1 -> DDM_CS&RC_Comparison/7
  DDM_CS&RC_Comparison/1 -> VHAL_FCM4CSErr_flg/1
  DDM_CS&RC_Comparison/2 -> VHAL_FCM4RCErr_flg/1
  [DT_CAN6_SG_FCM4] -> bus_selector1/1
  bus_selector1/1 -> ADASAngCtrlTqWeightGain/1(ADAS_AngCtrlTqWeightGain)  "<CAN6_ADAS_AngCtrlTqWeightGain>"
  ADASAngCtrlTqWeightGain/1(VHAL_ADASAngCtrlTqWeightGain_pct) -> VHAL_ADASAngCtrlTqWeightGain_pct/1
  [DT_CAN6_SG_FCM4] -> bus_selector2/1
  bus_selector2/1 -> ADASDesStrWhlAngCtrlCmd/1(ADAS_DesStrWhlAngCtrlCmd)  "<CAN6_ADAS_DesStrWhlAngCtrlCmd>"
  ADASDesStrWhlAngCtrlCmd/1(VHAL_ADASDesStrWhlAngCtrlCmd_Deg) -> VHAL_ADASDesStrWhlAngCtrlCmd_Deg/1
  [DT_CAN6_SG_FCM4] -> bus_selector3/1
  bus_selector3/1 -> ADASDrvInputTqBoostAct/1(ADAS_DrvInputTqBoostAct)  "<CAN6_ADAS_DrvInputTqBoostAct>"
  ADASDrvInputTqBoostAct/1(VHAL_ADASDrvInputTqBoostAct_flg) -> VHAL_ADASDrvInputTqBoostAct_flg/1
  [DT_CAN6_SG_FCM4] -> bus_selector4/1
  bus_selector4/1 -> ADASDrvInputTqBoostGain/1(ADAS_DrvInputTqBoostGain)  "<CAN6_ADAS_DrvInputTqBoostGain>"
  ADASDrvInputTqBoostGain/1(VHAL_ADASDrvInputTqBoostGain_pct) -> VHAL_ADASDrvInputTqBoostGain_pct/1
  [DT_CAN6_SG_FCM4] -> bus_selector5/1
  bus_selector5/1 -> ADASMaxAngCtrlOutTqLimit/1(ADAS_MaxAngCtrlOutTqLimit)  "<CAN6_ADAS_MaxAngCtrlOutTqLimit>"
  ADASMaxAngCtrlOutTqLimit/1(VHAL_ADASMaxAngCtrlOutTqLimit_Nm) -> VHAL_ADASMaxAngCtrlOutTqLimit_Nm/1
  [DT_CAN6_SG_FCM4] -> bus_selector6/1
  bus_selector6/1 -> ADASStrWhlAngCtrlStatus/1(ADAS_StrWhlAngCtrlStatus)  "<CAN6_ADAS_StrWhlAngCtrlStatus>"
  ADASStrWhlAngCtrlStatus/1(VHAL_ADASStrWhlAngCtrlStatus_flg) -> VHAL_ADASStrWhlAngCtrlStatus_flg/1

== system halin/HAL_IN/CAN6/SRR1 ==
  DT_CAN6_SG_SRR1 : Inport
  SRRBSDWarnL : Subsystem
  SRRBSDWarnR : Subsystem
  SRRODASoundL : Subsystem
  SRRODASoundR : Subsystem
  SRRODAWarnL : Subsystem
  SRRODAWarnR : Subsystem
  bus_selector : BusSelector  OutputSignals=CAN6_SRR_BSD_WarnL
  bus_selector1 : BusSelector  OutputSignals=CAN6_SRR_BSD_WarnR
  bus_selector2 : BusSelector  OutputSignals=CAN6_SRR_ODA_SoundL
  bus_selector3 : BusSelector  OutputSignals=CAN6_SRR_ODA_SoundR
  bus_selector4 : BusSelector  OutputSignals=CAN6_SRR_ODA_WarnL
  bus_selector5 : BusSelector  OutputSignals=CAN6_SRR_ODA_WarnR
  VHAL_SRRBSDWarnL_enum : Outport
  VHAL_SRRBSDWarnR_enum : Outport  Port=2
  VHAL_SRRODASoundL_flg : Outport  Port=3
  VHAL_SRRODASoundR_flg : Outport  Port=4
  VHAL_SRRODAWarnL_enum : Outport  Port=5
  VHAL_SRRODAWarnR_enum : Outport  Port=6
  wires:
  DT_CAN6_SG_SRR1/1 -> [DT_CAN6_SG_SRR1]
  [DT_CAN6_SG_SRR1] -> bus_selector/1
  bus_selector/1 -> SRRBSDWarnL/1(SRR_BSD_WarnL)  "<CAN6_SRR_BSD_WarnL>"
  SRRBSDWarnL/1(VHAL_SRRBSDWarnL_enum) -> VHAL_SRRBSDWarnL_enum/1
  [DT_CAN6_SG_SRR1] -> bus_selector1/1
  bus_selector1/1 -> SRRBSDWarnR/1(SRR_BSD_WarnR)  "<CAN6_SRR_BSD_WarnR>"
  SRRBSDWarnR/1(VHAL_SRRBSDWarnR_enum) -> VHAL_SRRBSDWarnR_enum/1
  [DT_CAN6_SG_SRR1] -> bus_selector2/1
  bus_selector2/1 -> SRRODASoundL/1(SRR_ODA_SoundL)  "<CAN6_SRR_ODA_SoundL>"
  SRRODASoundL/1(VHAL_SRRODASoundL_flg) -> VHAL_SRRODASoundL_flg/1
  [DT_CAN6_SG_SRR1] -> bus_selector3/1
  bus_selector3/1 -> SRRODASoundR/1(SRR_ODA_SoundR)  "<CAN6_SRR_ODA_SoundR>"
  SRRODASoundR/1(VHAL_SRRODASoundR_flg) -> VHAL_SRRODASoundR_flg/1
  [DT_CAN6_SG_SRR1] -> bus_selector4/1
  bus_selector4/1 -> SRRODAWarnL/1(SRR_ODA_WarnL)  "<CAN6_SRR_ODA_WarnL>"
  SRRODAWarnL/1(VHAL_SRRODAWarnL_enum) -> VHAL_SRRODAWarnL_enum/1
  [DT_CAN6_SG_SRR1] -> bus_selector5/1
  bus_selector5/1 -> SRRODAWarnR/1(SRR_ODA_WarnR)  "<CAN6_SRR_ODA_WarnR>"
  SRRODAWarnR/1(VHAL_SRRODAWarnR_enum) -> VHAL_SRRODAWarnR_enum/1

== system halin/HAL_IN/CAN6/VHAL_CANMsgInvalidFCM1_flg ==
  Cast To Boolean13 : DataTypeConversion  OutDataTypeStr=boolean
  Constant : Constant  Value=TRUE
  Latch13 : hcu_lib/Basic_Blocks/Latch
  Switch13 : Switch  Criteria=u2 ~= 0
  Unit Delay : UnitDelay  SampleTime=-1  HasFrameUpgradeWarning=on
  UnitConverter : DataTypeConversion  OutDataTypeStr=boolean
  Out : Outport
  wires:
  Constant/1 -> Switch13/3
  Unit Delay/1 -> Cast To Boolean13/1
  Cast To Boolean13/1 -> Switch13/1, Latch13/1
  Switch13/1 -> UnitConverter/1
  Latch13/1 -> Switch13/2
  UnitConverter/1 -> Unit Delay/1, Out/1  "VHAL_CANMsgInvalidFCM1_flg"

== system halin/HAL_IN/CAN6/VHAL_CANMsgInvalidFCM2_flg ==
  Cast To Boolean13 : DataTypeConversion  OutDataTypeStr=boolean
  Constant : Constant  Value=TRUE
  Latch13 : hcu_lib/Basic_Blocks/Latch
  Switch13 : Switch  Criteria=u2 ~= 0
  Unit Delay : UnitDelay  SampleTime=-1  HasFrameUpgradeWarning=on
  UnitConverter : DataTypeConversion  OutDataTypeStr=boolean
  Out : Outport
  wires:
  Constant/1 -> Switch13/3
  Unit Delay/1 -> Cast To Boolean13/1
  Cast To Boolean13/1 -> Switch13/1, Latch13/1
  Switch13/1 -> UnitConverter/1
  Latch13/1 -> Switch13/2
  UnitConverter/1 -> Unit Delay/1, Out/1  "VHAL_CANMsgInvalidFCM2_flg"

== system halin/HAL_IN/CAN6/VHAL_CANMsgInvalidFCM3_flg ==
  Cast To Boolean13 : DataTypeConversion  OutDataTypeStr=boolean
  Constant : Constant  Value=TRUE
  Latch13 : hcu_lib/Basic_Blocks/Latch
  Switch13 : Switch  Criteria=u2 ~= 0
  Unit Delay : UnitDelay  SampleTime=-1  HasFrameUpgradeWarning=on
  UnitConverter : DataTypeConversion  OutDataTypeStr=boolean
  Out : Outport
  wires:
  Constant/1 -> Switch13/3
  Unit Delay/1 -> Cast To Boolean13/1
  Cast To Boolean13/1 -> Switch13/1, Latch13/1
  Switch13/1 -> UnitConverter/1
  Latch13/1 -> Switch13/2
  UnitConverter/1 -> Unit Delay/1, Out/1  "VHAL_CANMsgInvalidFCM3_flg"

== system halin/HAL_IN/CAN6/VHAL_CANMsgInvalidFCM4_flg ==
  Cast To Boolean13 : DataTypeConversion  OutDataTypeStr=boolean
  Constant : Constant  Value=TRUE
  Latch13 : hcu_lib/Basic_Blocks/Latch
  Switch13 : Switch  Criteria=u2 ~= 0
  Unit Delay : UnitDelay  SampleTime=-1  HasFrameUpgradeWarning=on
  UnitConverter : DataTypeConversion  OutDataTypeStr=boolean
  Out : Outport
  wires:
  Constant/1 -> Switch13/3
  Unit Delay/1 -> Cast To Boolean13/1
  Cast To Boolean13/1 -> Switch13/1, Latch13/1
  Switch13/1 -> UnitConverter/1
  Latch13/1 -> Switch13/2
  UnitConverter/1 -> Unit Delay/1, Out/1  "VHAL_CANMsgInvalidFCM4_flg"

== system halin/HAL_IN/CAN6/VHAL_CANMsgInvalidSRR1_flg ==
  Cast To Boolean13 : DataTypeConversion  OutDataTypeStr=boolean
  Constant : Constant  Value=TRUE
  Latch13 : hcu_lib/Basic_Blocks/Latch
  Switch13 : Switch  Criteria=u2 ~= 0
  Unit Delay : UnitDelay  SampleTime=-1  HasFrameUpgradeWarning=on
  UnitConverter : DataTypeConversion  OutDataTypeStr=boolean
  Out : Outport
  wires:
  Constant/1 -> Switch13/3
  Unit Delay/1 -> Cast To Boolean13/1
  Cast To Boolean13/1 -> Switch13/1, Latch13/1
  Switch13/1 -> UnitConverter/1
  Latch13/1 -> Switch13/2
  UnitConverter/1 -> Unit Delay/1, Out/1  "VHAL_CANMsgInvalidSRR1_flg"

== system halin/HAL_IN/CAN1/ABM1/ABMPassengerODSSta ==
  ABM_Passenger_ODS_Sta : Inport
  UnitConverter : DataTypeConversion  OutDataTypeStr=uint8
  VHAL_ABMPassengerODSSta_flg : Outport
  wires:
  UnitConverter/1 -> VHAL_ABMPassengerODSSta_flg/1
  ABM_Passenger_ODS_Sta/1 -> UnitConverter/1

== system halin/HAL_IN/CAN1/ABM1/ABMRearPassengerCTRODSSta ==
  ABM_RearPassengerCTR_ODS_Sta : Inport
  UnitConverter : DataTypeConversion  OutDataTypeStr=uint8
  VHAL_ABMRearPassengerCTRODSSta_flg : Outport
  wires:
  UnitConverter/1 -> VHAL_ABMRearPassengerCTRODSSta_flg/1
  ABM_RearPassengerCTR_ODS_Sta/1 -> UnitConverter/1

== system halin/HAL_IN/CAN1/ABM1/ABMRearPassengerLHODSSta ==
  ABM_RearPassengerLH_ODS_Sta : Inport
  UnitConverter : DataTypeConversion  OutDataTypeStr=uint8
  VHAL_ABMRearPassengerLHODSSta_flg : Outport
  wires:
  UnitConverter/1 -> VHAL_ABMRearPassengerLHODSSta_flg/1
  ABM_RearPassengerLH_ODS_Sta/1 -> UnitConverter/1

== system halin/HAL_IN/CAN1/ABM1/ABMRearPassengerRHODSSta ==
  ABM_RearPassengerRH_ODS_Sta : Inport
  UnitConverter : DataTypeConversion  OutDataTypeStr=uint8
  VHAL_ABMRearPassengerRHODSSta_flg : Outport
  wires:
  UnitConverter/1 -> VHAL_ABMRearPassengerRHODSSta_flg/1
  ABM_RearPassengerRH_ODS_Sta/1 -> UnitConverter/1

== system halin/HAL_IN/CAN1/ABM1/AirBagFailCmd ==
  AirBagFailCmd : Inport
  UnitConverter : DataTypeConversion  OutDataTypeStr=uint8
  VHAL_AirBagFailCmd_flg : Outport
  wires:
  UnitConverter/1 -> VHAL_AirBagFailCmd_flg/1
  AirBagFailCmd/1 -> UnitConverter/1

== system halin/HAL_IN/CAN1/ABM1/ChecksumABM1 ==
  Checksum_ABM1 : Inport
  UnitConverter : DataTypeConversion  OutDataTypeStr=uint8
  VHAL_ChecksumABM1_enum : Outport
  wires:
  UnitConverter/1 -> VHAL_ChecksumABM1_enum/1
  Checksum_ABM1/1 -> UnitConverter/1

== system halin/HAL_IN/CAN1/ABM1/CrashOutputSts ==
  CrashOutputSts : Inport
  UnitConverter : DataTypeConversion  OutDataTypeStr=uint8
  VHAL_CrashOutputSts_enum : Outport
  wires:
  UnitConverter/1 -> VHAL_CrashOutputSts_enum/1
  CrashOutputSts/1 -> UnitConverter/1

== system halin/HAL_IN/CAN1/ABM1/DriverSeatBeltCmd ==
  DriverSeatBeltCmd : Inport
  UnitConverter : DataTypeConversion  OutDataTypeStr=uint8
  VHAL_DriverSeatBeltCmd_flg : Outport
  wires:
  UnitConverter/1 -> VHAL_DriverSeatBeltCmd_flg/1
  DriverSeatBeltCmd/1 -> UnitConverter/1

== system halin/HAL_IN/CAN1/ABM1/LifeCountABM1 ==
  LifeCount_ABM1 : Inport
  UnitConverter : DataTypeConversion  OutDataTypeStr=uint8
  VHAL_LifeCountABM1_enum : Outport
  wires:
  UnitConverter/1 -> VHAL_LifeCountABM1_enum/1
  LifeCount_ABM1/1 -> UnitConverter/1

== system halin/HAL_IN/CAN1/ABM1/PABSwitchCmd ==
  PABSwitchCmd : Inport
  UnitConverter : DataTypeConversion  OutDataTypeStr=uint8
  VHAL_PABSwitchCmd_flg : Outport
  wires:
  UnitConverter/1 -> VHAL_PABSwitchCmd_flg/1
  PABSwitchCmd/1 -> UnitConverter/1

== system halin/HAL_IN/CAN1/ABM1/PsngrSeatBeltCmd ==
  PsngrSeatBeltCmd : Inport
  UnitConverter : DataTypeConversion  OutDataTypeStr=uint8
  VHAL_PsngrSeatBeltCmd_flg : Outport
  wires:
  UnitConverter/1 -> VHAL_PsngrSeatBeltCmd_flg/1
  PsngrSeatBeltCmd/1 -> UnitConverter/1

== system halin/HAL_IN/CAN1/ABM1/RCenterSeatBeltCmd ==
  RCenterSeatBeltCmd : Inport
  UnitConverter : DataTypeConversion  OutDataTypeStr=uint8
  VHAL_RCenterSeatBeltCmd_flg : Outport
  wires:
  UnitConverter/1 -> VHAL_RCenterSeatBeltCmd_flg/1
  RCenterSeatBeltCmd/1 -> UnitConverter/1

== system halin/HAL_IN/CAN1/ABM1/RDriverSeatBeltCmd ==
  RDriverSeatBeltCmd : Inport
  UnitConverter : DataTypeConversion  OutDataTypeStr=uint8
  VHAL_RDriverSeatBeltCmd_flg : Outport
  wires:
  UnitConverter/1 -> VHAL_RDriverSeatBeltCmd_flg/1
  RDriverSeatBeltCmd/1 -> UnitConverter/1

== system halin/HAL_IN/CAN1/ABM1/RPsngrSeatBeltCmd ==
  RPsngrSeatBeltCmd : Inport
  UnitConverter : DataTypeConversion  OutDataTypeStr=uint8
  VHAL_RPsngrSeatBeltCmd_flg : Outport
  wires:
  UnitConverter/1 -> VHAL_RPsngrSeatBeltCmd_flg/1
  RPsngrSeatBeltCmd/1 -> UnitConverter/1

== system halin/HAL_IN/CAN1/ABM1/TLHPsngrSeatBeltCmd ==
  TLHPsngrSeatBeltCmd : Inport
  UnitConverter : DataTypeConversion  OutDataTypeStr=uint8
  VHAL_TLHPsngrSeatBeltCmd_flg : Outport
  wires:
  UnitConverter/1 -> VHAL_TLHPsngrSeatBeltCmd_flg/1
  TLHPsngrSeatBeltCmd/1 -> UnitConverter/1

== system halin/HAL_IN/CAN1/ABM1/TRHPsngrSeatBeltCmd ==
  TRHPsngrSeatBeltCmd : Inport
  UnitConverter : DataTypeConversion  OutDataTypeStr=uint8
  VHAL_TRHPsngrSeatBeltCmd_flg : Outport
  wires:
  UnitConverter/1 -> VHAL_TRHPsngrSeatBeltCmd_flg/1
  TRHPsngrSeatBeltCmd/1 -> UnitConverter/1

== system halin/HAL_IN/CAN1/EPB1/DOASta ==
  DOA_Sta : Inport
  UnitConverter : DataTypeConversion  OutDataTypeStr=uint8
  VHAL_DOASta_flg : Outport
  wires:
  UnitConverter/1 -> VHAL_DOASta_flg/1
  DOA_Sta/1 -> UnitConverter/1

== system halin/HAL_IN/CAN1/EPB1/EPB1RC ==
  EPB1_RC : Inport
  UnitConverter : DataTypeConversion  OutDataTypeStr=uint8
  VHAL_EPB1RC_enum : Outport
  wires:
  UnitConverter/1 -> VHAL_EPB1RC_enum/1
  EPB1_RC/1 -> UnitConverter/1

== system halin/HAL_IN/CAN1/EPB1/EPBCarWashMode ==
  EPBCarWashMode : Inport
  UnitConverter : DataTypeConversion  OutDataTypeStr=uint8
  VHAL_EPBCarWashMode_flg : Outport
  wires:
  UnitConverter/1 -> VHAL_EPBCarWashMode_flg/1
  EPBCarWashMode/1 -> UnitConverter/1

== system halin/HAL_IN/CAN1/EPB1/EPBErrSta ==
  EPBErrSta : Inport
  UnitConverter : DataTypeConversion  OutDataTypeStr=uint8
  VHAL_EPBErrSta_enum : Outport
  wires:
  UnitConverter/1 -> VHAL_EPBErrSta_enum/1
  EPBErrSta/1 -> UnitConverter/1

== system halin/HAL_IN/CAN1/EPB1/EPBExtApplyAvail ==
  EPBExtApplyAvail : Inport
  UnitConverter : DataTypeConversion  OutDataTypeStr=uint8
  VHAL_EPBExtApplyAvail_flg : Outport
  wires:
  UnitConverter/1 -> VHAL_EPBExtApplyAvail_flg/1
  EPBExtApplyAvail/1 -> UnitConverter/1

== system halin/HAL_IN/CAN1/EPB1/EPBExtReleaseAvail ==
  EPBExtReleaseAvail : Inport
  UnitConverter : DataTypeConversion  OutDataTypeStr=uint8
  VHAL_EPBExtReleaseAvail_flg : Outport
  wires:
  UnitConverter/1 -> VHAL_EPBExtReleaseAvail_flg/1
  EPBExtReleaseAvail/1 -> UnitConverter/1

== system halin/HAL_IN/CAN1/EPB1/EPBSta ==
  EPBSta : Inport
  UnitConverter : DataTypeConversion  OutDataTypeStr=uint8
  VHAL_EPBSta_enum : Outport
  wires:
  UnitConverter/1 -> VHAL_EPBSta_enum/1
  EPBSta/1 -> UnitConverter/1

== system halin/HAL_IN/CAN1/EPS1/DriIntend ==
  DriIntend : Inport
  UnitConverter : DataTypeConversion  OutDataTypeStr=uint8
  VHAL_DriIntend_enum : Outport
  wires:
  UnitConverter/1 -> VHAL_DriIntend_enum/1
  DriIntend/1 -> UnitConverter/1

== system halin/HAL_IN/CAN1/EPS1/EPSAOIControl ==
  EPS_AOI_Control : Inport
  UnitConverter : DataTypeConversion  OutDataTypeStr=uint8
  VHAL_EPSAOIControl_enum : Outport
  wires:
  UnitConverter/1 -> VHAL_EPSAOIControl_enum/1
  EPS_AOI_Control/1 -> UnitConverter/1

== system halin/HAL_IN/CAN1/EPS1/EPSRC ==
  EPS_RC : Inport
  UnitConverter : DataTypeConversion  OutDataTypeStr=uint8
  VHAL_EPSRC_enum : Outport
  wires:
  UnitConverter/1 -> VHAL_EPSRC_enum/1
  EPS_RC/1 -> UnitConverter/1

== system halin/HAL_IN/CAN1/EPS1/EPSTOIActivation ==
  EPS_TOI_Activation : Inport
  UnitConverter : DataTypeConversion  OutDataTypeStr=uint8
  VHAL_EPSTOIActivation_flg : Outport
  wires:
  UnitConverter/1 -> VHAL_EPSTOIActivation_flg/1
  EPS_TOI_Activation/1 -> UnitConverter/1

== system halin/HAL_IN/CAN1/EPS1/EPSTOIFault ==
  EPS_TOI_Fault : Inport
  UnitConverter : DataTypeConversion  OutDataTypeStr=uint8
  VHAL_EPSTOIFault_flg : Outport
  wires:
  UnitConverter/1 -> VHAL_EPSTOIFault_flg/1
  EPS_TOI_Fault/1 -> UnitConverter/1

== system halin/HAL_IN/CAN1/EPS1/EPSTOIUnavailable ==
  EPS_TOI_Unavailable : Inport
  UnitConverter : DataTypeConversion  OutDataTypeStr=uint8
  VHAL_EPSTOIUnavailable_flg : Outport
  wires:
  UnitConverter/1 -> VHAL_EPSTOIUnavailable_flg/1
  EPS_TOI_Unavailable/1 -> UnitConverter/1

== system halin/HAL_IN/CAN1/EPS1/EpasFailed ==
  EpasFailed : Inport
  UnitConverter : DataTypeConversion  OutDataTypeStr=uint8
  VHAL_EpasFailed_enum : Outport
  wires:
  UnitConverter/1 -> VHAL_EpasFailed_enum/1
  EpasFailed/1 -> UnitConverter/1
